simulink model "sim_lab5"  (R2020b)
settings: Solver=FixedStepAuto  StartTime=0.0  StopTime=10  FixedStep=0.0001  RelTol=1e-3
values from neighbouring files (symbols this model uses):
  cont_model = tf ( c_nom , c_denom )    [Copy_of_zadanie2.m]    (also in laboratorium5.m; zadanie2.m)
  disc_model = c2d( cont_model, Ts )    [laboratorium5.m]    (also in zadanie2.m)
  final_value = 1    [Copy_of_zadanie2.m]    (also in laboratorium5.m; zadanie2.m)
  init_value = 0    [Copy_of_zadanie2.m]    (also in laboratorium5.m; zadanie2.m)
  time_step = 0    [Copy_of_zadanie2.m]    (also in laboratorium5.m; zadanie2.m)
  Ts = 0.1    [laboratorium5.m]    (also in zadanie2.m)
settings Model: Creator=student  LastModifiedBy=student

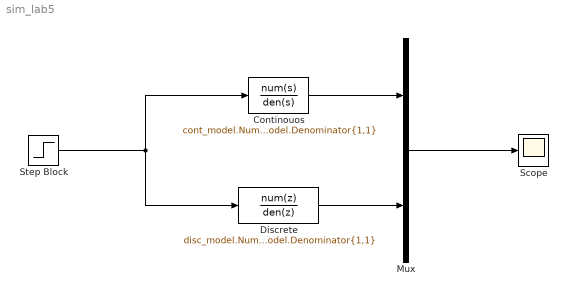
== system sim_lab5 ==
  Continouos : TransferFcn  Numerator=cont_model.Numerator{1,1}  Denominator=cont_model.Denominator{1,1}
  Discrete : DiscreteTransferFcn  Numerator=disc_model.Numerator{1,1}  Denominator=disc_model.Denominator{1,1}  SampleTime=Ts
  Mux : Mux  Inputs=2
  Scope : Scope
  Step Block : Step  Time=time_step  Before=init_value  After=final_value  SampleTime=0
  wires:
  Step Block/1 -> Discrete/1, Continouos/1
  Continouos/1 -> Mux/1
  Discrete/1 -> Mux/2
  Mux/1 -> Scope/1
